simulink model "pres_ctrl_design"  (R2021b)
settings: Solver=VariableStepAuto  StartTime=0.0  StopTime=simlegth  RelTol=1e-3
values from neighbouring files (symbols this model uses):
  Ad = [cos(w*ts) sin(w*ts)/w; -w*sin(w*ts) cos(w*ts)]    [pres_ctrl_design_init.m]
  Bd = [(1-cos(w*ts))/w^2 sin(w*ts)/w]'    [pres_ctrl_design_init.m]
  C = [0 1]    [pres_ctrl_design_init.m]
  ki = 18    [pres_ctrl_design_init.m]
  kp = ki/omega_c    (= 0.45)    [pres_ctrl_design_init.m]
  L = 1e-3    (= 0.001)    [pres_ctrl_design_init.m]
  R = 1e-2    (= 0.01)    [pres_ctrl_design_init.m]
  Tc = ts/20    (= 5e-05)    [pres_ctrl_design_init.m]
  ts = 1e-3    (= 0.001)    [pres_ctrl_design_init.m]
  w = 2*pi*50    (= 314.159265359)    [pres_ctrl_design_init.m]
libraries: cstblocks x1
settings Model: Creator=dabagnara  LastModifiedBy=dbagn
settings SolverCC: AlgebraicLoopSolver=TrustRegion
settings DataIOCC: ReturnWorkspaceOutputs=off
settings DebuggingCC: SFMachineParentedDataDiag=warning

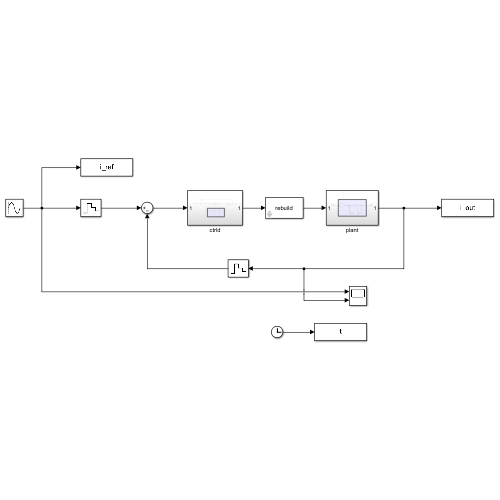
[thumbnail: Simulink's stored preview of the top-level diagram]
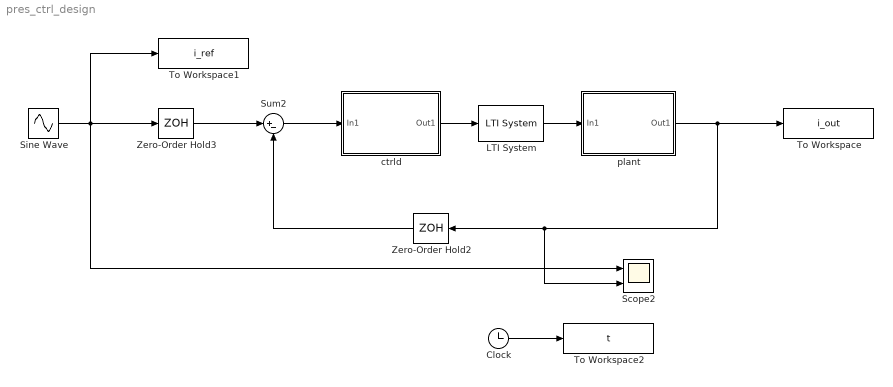
== system pres_ctrl_design ==
  Clock : Clock
  LTI System : cstblocks/LTI System  sys=rebuild  IC=[]
  Scope2 : Scope  NumInputPorts=2
  Sine Wave : Sin  Frequency=w  Phase=pi/2  SampleTime=0
  Sum2 : Sum  Inputs=|+-
  To Workspace : ToWorkspace  VariableName=i_out  SampleTime=Tc
  To Workspace1 : ToWorkspace  VariableName=i_ref  SampleTime=Tc
  To Workspace2 : ToWorkspace  VariableName=t  SampleTime=Tc
  Zero-Order Hold2 : ZeroOrderHold  SampleTime=ts
  Zero-Order Hold3 : ZeroOrderHold  SampleTime=ts
  ctrld : Subsystem
  plant : Subsystem
  wires:
  Zero-Order Hold3/1 -> Sum2/1
  Zero-Order Hold2/1 -> Sum2/2
  Sine Wave/1 -> Zero-Order Hold3/1, To Workspace1/1, Scope2/1
  Sum2/1 -> ctrld/1(In1)
  Clock/1 -> To Workspace2/1
  ctrld/1(Out1) -> LTI System/1
  plant/1(Out1) -> Scope2/2, Zero-Order Hold2/1, To Workspace/1
  LTI System/1 -> plant/1(In1)

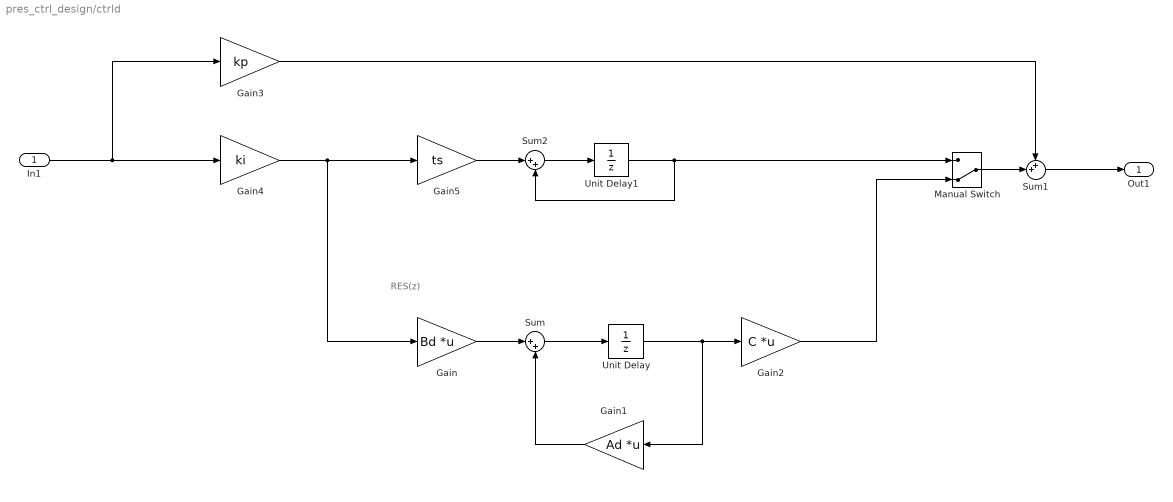
== system pres_ctrl_design/ctrld ==
  note: RES(z)
  In1 : Inport
  Gain : Gain  Gain=Bd  Multiplication=Matrix(K*u)
  Gain1 : Gain  Gain=Ad  Multiplication=Matrix(K*u)
  Gain2 : Gain  Gain=C  Multiplication=Matrix(K*u)
  Gain3 : Gain  Gain=kp
  Gain4 : Gain  Gain=ki
  Gain5 : Gain  Gain=ts
  Manual Switch : ManualSwitch  CurrentSetting=0
  Sum : Sum  Inputs=|++
  Sum1 : Sum  Inputs=++|
  Sum2 : Sum  Inputs=|++
  Unit Delay : UnitDelay  SampleTime=ts  HasFrameUpgradeWarning=on
  Unit Delay1 : UnitDelay  SampleTime=ts  HasFrameUpgradeWarning=on
  Out1 : Outport
  wires:
  In1/1 -> Gain4/1, Gain3/1
  Sum/1 -> Unit Delay/1
  Gain/1 -> Sum/1
  Gain1/1 -> Sum/2
  Unit Delay/1 -> Gain2/1, Gain1/1
  Gain4/1 -> Gain5/1, Gain/1
  Sum1/1 -> Out1/1
  Gain3/1 -> Sum1/1
  Manual Switch/1 -> Sum1/2
  Gain2/1 -> Manual Switch/2
  Unit Delay1/1 -> Sum2/2, Manual Switch/1
  Sum2/1 -> Unit Delay1/1
  Gain5/1 -> Sum2/1

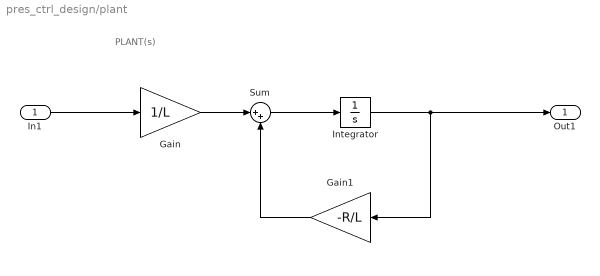
== system pres_ctrl_design/plant ==
  note: PLANT(s)
  In1 : Inport
  Gain : Gain  Gain=1/L
  Gain1 : Gain  Gain=-R/L
  Integrator : Integrator
  Sum : Sum  Inputs=|++
  Out1 : Outport
  wires:
  Gain1/1 -> Sum/2
  In1/1 -> Gain/1
  Sum/1 -> Integrator/1
  Integrator/1 -> Out1/1, Gain1/1
  Gain/1 -> Sum/1
